simulink model "Fusion_Frame_Model_Architecture"  (R2018a)
settings: Solver=FixedStepAuto  StartTime=0.0  StopTime=SimulationTime  FixedStep=SamplingTime  RelTol=1e-3
undefined symbols (not defined in the file or in its folder): ACTIVATE_CAM, ACTIVATE_RAD, CAM1_detTimeStamp, CAM1_MeasNoise, CAM1_objClassID, CAM1_PX, CAM1_PY, CAM1_VX, CAM1_VY, CAM2_detTimeStamp, CAM2_MeasNoise, CAM2_objClassID, CAM2_PX, CAM2_PY, CAM2_VX, CAM2_VY, CAM3_detTimeStamp, CAM3_MeasNoise, CAM3_objClassID, CAM3_PX, CAM3_PY, CAM3_VX, CAM3_VY, CAM4_detTimeStamp, CAM4_MeasNoise, CAM4_objClassID, CAM4_PX, CAM4_PY, CAM4_VX, CAM4_VY, CAM5_detTimeStamp, CAM5_MeasNoise, CAM5_objClassID, CAM5_PX, CAM5_PY, CAM5_VX, CAM5_VY, CAM6_detTimeStamp, CAM6_MeasNoise, CAM6_objClassID, CAM6_PX, CAM6_PY, CAM6_VX, CAM6_VY, CAM7_detTimeStamp, CAM7_MeasNoise, CAM7_objClassID, CAM7_PX, CAM7_PY, CAM7_VX, CAM7_VY, CAM8_detTimeStamp, CAM8_MeasNoise, CAM8_objClassID, CAM8_PX, CAM8_PY, CAM8_VX, CAM8_VY, CAM_nMeas, CAM_TYPE ... (+181)
libraries: simulink_extras x4
(part 9 of 11)

== system Fusion_Frame_Model_Architecture/SENSOR_FUSION_SYSTEM/OBJECT_TRACKER_SENSOR_FUSION/RADAR_HOMOGENEOUS_FUSION/SIMPLYFIED_DBSCAN_FOR_RADAR_MEASUREMENT_GROUPING/DBSCAN_MEASUREMENT_GROUPING/COMPUTE_MEAN_IF_CLUSTER_FORMED/COMPUTE_MEAN_SUM ==
  ClusterMembers : Inport
  nPoints : Inport  Port=2
  MeasArray : Inport  Port=3
  Add1 : Sum
  Bus Selector : BusSelector  OutputSignals=MeasArray
  For Iterator : ForIterator  ResetStates=reset  IterationSource=external
  Selector : Selector  NumberOfDimensions=2  InputPortWidth=3  IndexOptions=Select all,Index vector (port)  Indices=[1 3],1  OutputSizes=1,1
  Selector1 : Selector  NumberOfDimensions=2  InputPortWidth=3  IndexOptions=Select all,Index vector (port)  Indices=[1 3],1  OutputSizes=1,1
  Unit Delay : UnitDelay  InitialCondition=single(0)  SampleTime=-1
  ClusterMeanSUM : Outport
  wires:
  nPoints/1 -> For Iterator/1
  ClusterMembers/1 -> Selector/1
  For Iterator/1 -> Selector/2
  MeasArray/1 -> Bus Selector/1
  Bus Selector/1 -> Selector1/1  "<MeasArray>"
  Selector/1 -> Selector1/2
  Selector1/1 -> Add1/2
  Unit Delay/1 -> Add1/1
  Add1/1 -> ClusterMeanSUM/1, Unit Delay/1

== system Fusion_Frame_Model_Architecture/SENSOR_FUSION_SYSTEM/OBJECT_TRACKER_SENSOR_FUSION/RADAR_HOMOGENEOUS_FUSION/SIMPLYFIED_DBSCAN_FOR_RADAR_MEASUREMENT_GROUPING/DBSCAN_MEASUREMENT_GROUPING/COMPUTE_MEAN_IF_CLUSTER_FORMED/GET_DATA ==
  CLSTR : Inport
  Bus Selector : BusSelector  OutputSignals=ClusterSizes,nClusters,ClusterMember
  Selector : Selector  NumberOfDimensions=2  InputPortWidth=3  IndexOptions=Select all,Index vector (port)  Indices=[1 3],1  OutputSizes=1,1
  nPts : Outport
  <ClusterMember> : Outport  Port=2
  wires:
  Bus Selector/1 -> Selector/1  "<ClusterSizes>"
  Selector/1 -> nPts/1
  Bus Selector/2 -> Selector/2  "<nClusters>"
  Bus Selector/3 -> <ClusterMember>/1  "<ClusterMember>"
  CLSTR/1 -> Bus Selector/1

== system Fusion_Frame_Model_Architecture/SENSOR_FUSION_SYSTEM/OBJECT_TRACKER_SENSOR_FUSION/RADAR_HOMOGENEOUS_FUSION/SIMPLYFIED_DBSCAN_FOR_RADAR_MEASUREMENT_GROUPING/DBSCAN_MEASUREMENT_GROUPING/FORM_CLUSTER/CHECK_CONDITION ==
  idx_i : Inport
  CLSTR_in : Inport  Port=2
  Bus Selector : BusSelector  OutputSignals=isMeasVisitedFlag
  Logical Operator1 : Logic  Operator=NOT  AllPortsSameDT=off  OutDataTypeStr=boolean
  Selector1 : Selector  NumberOfDimensions=2  InputPortWidth=3  IndexOptions=Select all,Index vector (port)  Indices=1,1  OutputSizes=1,1
  Unit Delay : UnitDelay  InitialCondition=CLSTR_SNSR_DELAY_INIT  SampleTime=-1
  isNotVisited : Outport
  CLSTR_out : Outport  Port=2
  wires:
  Logical Operator1/1 -> isNotVisited/1
  Selector1/1 -> Logical Operator1/1
  idx_i/1 -> Selector1/2
  CLSTR_in/1 -> Unit Delay/1
  Bus Selector/1 -> Selector1/1  "<isMeasVisitedFlag>"
  Unit Delay/1 -> CLSTR_out/1, Bus Selector/1

== system Fusion_Frame_Model_Architecture/SENSOR_FUSION_SYSTEM/OBJECT_TRACKER_SENSOR_FUSION/RADAR_HOMOGENEOUS_FUSION/SIMPLYFIED_DBSCAN_FOR_RADAR_MEASUREMENT_GROUPING/DBSCAN_MEASUREMENT_GROUPING/FORM_CLUSTER/DBSCAN ==
  CLSTR_DATA : Inport
  measArray : Inport  Port=2
  idx_i : Inport  Port=3
  Action Port : ActionPort  ActionType=then
  DBSCAN_PROPAGATE_AND_EXPAND_CLUSTER : Subsystem
  INITIALIZE_CLUSTER : Subsystem
  Subsystem : Subsystem
  nPtsEps : Outport
  CLSTR_DATA_UPD : Outport  Port=2
  wires:
  idx_i/1 -> INITIALIZE_CLUSTER/3(idx_i)
  INITIALIZE_CLUSTER/2(CLUSTER_DATA) -> DBSCAN_PROPAGATE_AND_EXPAND_CLUSTER/3(CLSTR_DATA)
  INITIALIZE_CLUSTER/1(nRadMeas) -> DBSCAN_PROPAGATE_AND_EXPAND_CLUSTER/1(nMeas)
  CLSTR_DATA/1 -> INITIALIZE_CLUSTER/1(CLUSTERING_DATA)
  [meas] -> DBSCAN_PROPAGATE_AND_EXPAND_CLUSTER/2(measArray)
  measArray/1 -> INITIALIZE_CLUSTER/2(RAD_MEAS_CTS), [meas]
  DBSCAN_PROPAGATE_AND_EXPAND_CLUSTER/1(CLSTR_DATA_UPD) -> CLSTR_DATA_UPD/1, Subsystem/1(CLSTR_DATA)
  Subsystem/1(ClstrSize) -> nPtsEps/1

== system Fusion_Frame_Model_Architecture/SENSOR_FUSION_SYSTEM/OBJECT_TRACKER_SENSOR_FUSION/RADAR_HOMOGENEOUS_FUSION/SIMPLYFIED_DBSCAN_FOR_RADAR_MEASUREMENT_GROUPING/DBSCAN_MEASUREMENT_GROUPING/FORM_CLUSTER/MERGE_SIGNALS ==
  CLSTR_NO_UPD : Inport
  nPtsEpsNoUpd : Inport  Port=2
  nPtsUpd : Inport  Port=3
  CLSTR_UPD : Inport  Port=4
  Merge : Merge
  Merge1 : Merge
  nPtsEps : Outport
  CLSTR_DATA : Outport  Port=2
  wires:
  CLSTR_NO_UPD/1 -> Merge1/1
  Merge1/1 -> CLSTR_DATA/1
  nPtsEpsNoUpd/1 -> Merge/1
  Merge/1 -> nPtsEps/1
  nPtsUpd/1 -> Merge/2
  CLSTR_UPD/1 -> Merge1/2

== system Fusion_Frame_Model_Architecture/SENSOR_FUSION_SYSTEM/OBJECT_TRACKER_SENSOR_FUSION/RADAR_HOMOGENEOUS_FUSION/SIMPLYFIED_DBSCAN_FOR_RADAR_MEASUREMENT_GROUPING/DBSCAN_MEASUREMENT_GROUPING/FORM_CLUSTER/NO_CLUSTER_FORMED ==
  CLSTR_DATA : Inport
  Action Port : ActionPort  ActionType=else
  Constant : Constant  Value=uint16(0)
  CLSTR_DATA_NO_UPD : Outport
  nPtsEpsNoUpd : Outport  Port=2
  wires:
  CLSTR_DATA/1 -> CLSTR_DATA_NO_UPD/1
  Constant/1 -> nPtsEpsNoUpd/1

== system Fusion_Frame_Model_Architecture/SENSOR_FUSION_SYSTEM/OBJECT_TRACKER_SENSOR_FUSION/RADAR_HOMOGENEOUS_FUSION/SIMPLYFIED_DBSCAN_FOR_RADAR_MEASUREMENT_GROUPING/DBSCAN_MEASUREMENT_GROUPING/MERGE_SIGNALS/GET_DATA_FROM_BUS ==
  CLSTR_DATA : Inport
  Bus Selector : BusSelector  OutputSignals=ClusterCenter,ClusterCovariance,nClusters
  <ClusterCenter> : Outport
  <ClusterCovariance> : Outport  Port=2
  <nClusters> : Outport  Port=3
  wires:
  Bus Selector/3 -> <nClusters>/1  "<nClusters>"
  Bus Selector/1 -> <ClusterCenter>/1  "<ClusterCenter>"
  CLSTR_DATA/1 -> Bus Selector/1
  Bus Selector/2 -> <ClusterCovariance>/1  "<ClusterCovariance>"

== system Fusion_Frame_Model_Architecture/SENSOR_FUSION_SYSTEM/OBJECT_TRACKER_SENSOR_FUSION/RADAR_HOMOGENEOUS_FUSION/SIMPLYFIED_DBSCAN_FOR_RADAR_MEASUREMENT_GROUPING/DBSCAN_MEASUREMENT_GROUPING/MERGE_SIGNALS/SET_DATA_TO_BUS ==
  CLSTR_DATA : Inport
  Mean_ARRAY : Inport  Port=2
  Cov_ARRAY : Inport  Port=3
  Bus Creator : BusCreator  Inputs=7  OutDataTypeStr=Bus: CLUSTER_DATA_STRUCT_SNSR  NonVirtualBus=on
      settings: InheritFromInputs=off
  Bus Selector1 : BusSelector  OutputSignals=ClusterCenter,ClusterCovariance,ClusterSizes,ClusterToMeasAssignment,isMeasVisitedFlag,nClusters,ClusterMember
  Constant1 : Constant  Value=ClusterMemArray_SNSR
  Reshape1 : Reshape  OutputDimensionality=Row vector (2-D)
  Terminator1 : Terminator
  Terminator2 : Terminator
  Terminator3 : Terminator
  "CLSTR_DATA_UPD " : Outport
  wires:
  Constant1/1 -> Reshape1/1  "ClusterMember"
  Bus Selector1/5 -> Bus Creator/5  "<isMeasVisitedFlag>"
  Cov_ARRAY/1 -> Bus Creator/2  "ClusterCovariance"
  Mean_ARRAY/1 -> Bus Creator/1  "ClusterCenter"
  Bus Selector1/1 -> Terminator2/1  "<ClusterCenter>"
  Bus Selector1/7 -> Terminator1/1  "<ClusterMember>"
  Bus Selector1/2 -> Terminator3/1  "<ClusterCovariance>"
  Bus Selector1/3 -> Bus Creator/3  "<ClusterSizes>"
  Reshape1/1 -> Bus Creator/7  "ClusterMember"
  Bus Selector1/4 -> Bus Creator/4  "<ClusterToMeasAssignment>"
  Bus Selector1/6 -> Bus Creator/6  "<nClusters>"
  Bus Creator/1 -> "CLSTR_DATA_UPD "/1
  CLSTR_DATA/1 -> Bus Selector1/1

== system Fusion_Frame_Model_Architecture/SENSOR_FUSION_SYSTEM/OBJECT_TRACKER_SENSOR_FUSION/RADAR_HOMOGENEOUS_FUSION/SIMPLYFIED_DBSCAN_FOR_RADAR_MEASUREMENT_GROUPING/DBSCAN_MEASUREMENT_GROUPING/MERGE_SIGNALS/UPDATE_CLUSTER_DATA ==
  Center_ARRAY : Inport
  Cov_ARRAY : Inport  Port=2
  ID : Inport  Port=3
  mean1 : Inport  Port=4
  mean2 : Inport  Port=5
  Cov1 : Inport  Port=6
  Cov2 : Inport  Port=7
  FLAG : Inport  Port=8
  Assignment : Assignment  NumberOfDimensions=2  DiagnosticForDimensions=Warning  IndexOptions=Assign all,Index vector (port)  Indices=1,1  OutputSizes=1,1
  Assignment1 : Assignment  NumberOfDimensions=3  DiagnosticForDimensions=Warning  IndexOptions=Assign all,Assign all,Index vector (port)  Indices=1,1,1  OutputSizes=1,1,1
  Merge : Merge
  Merge2 : Merge
  Selector : Selector  NumberOfDimensions=2  InputPortWidth=3  IndexOptions=Select all,Index vector (port)  Indices=[1 3],1  OutputSizes=1,1
  Selector1 : Selector  NumberOfDimensions=3  InputPortWidth=3  IndexOptions=Select all,Select all,Index vector (port)  Indices=[1 3],1,1  OutputSizes=1,1,1
  Switch : Switch  Criteria=u2 ~= 0
  Switch1 : Switch  Criteria=u2 ~= 0
  CenterUpd : Outport
  CovUpd : Outport  Port=2
  wires:
  Selector/1 -> Switch/3
  Merge2/1 -> Switch1/1
  Cov_ARRAY/1 -> Assignment1/1, Selector1/1
  mean1/1 -> Merge/1
  Selector1/1 -> Switch1/3
  Merge/1 -> Switch/1
  Switch1/1 -> Assignment1/2
  Switch/1 -> Assignment/2
  Cov2/1 -> Merge2/2
  Assignment1/1 -> CovUpd/1
  Assignment/1 -> CenterUpd/1
  Cov1/1 -> Merge2/1
  mean2/1 -> Merge/2
  FLAG/1 -> [FLAG]
  [FLAG] -> Switch/2
  [FLAG] -> Switch1/2
  [ID] -> Assignment/3, Selector/2
  ID/1 -> [ID], Assignment1/3, Selector1/2
  Center_ARRAY/1 -> Selector/1, Assignment/1

== system Fusion_Frame_Model_Architecture/SENSOR_FUSION_SYSTEM/OBJECT_TRACKER_SENSOR_FUSION/SENSOR_LAYOUT_AND_CHRACTERIZATION/PRE_COMPUTE_SENSOR_FOV_GRID/COMPUTE_CAMERA_SNSR_GRID/ComputeCoverageANDConfidence/Compute_Cell_X_and_Y_index ==
  CellIndex : Inport
  GridID_vec : Inport  Port=2
  GridParam : Inport  Port=3
  SensorExtrinsicParam : Inport  Port=4
  SensorIntrinsicParam : Inport  Port=5
  Compute_Cell_X_Y_Center_Coordinate : Subsystem
  Compute_FOV_Overlap_with_Cell_and_Region_Confidence : Subsystem
  GET_DATA : Subsystem
  Transform_Cell_Coordinate_Vehicle_Frame_To_Sensor_Frame : Subsystem
  RegionConfidence : Outport
  FOVOverlap : Outport  Port=2
  wires:
  GridID_vec/1 -> GET_DATA/1(GridID_vector)
  CellIndex/1 -> GET_DATA/2(index)
  GridParam/1 -> GET_DATA/3(GridParam)
  GET_DATA/1(CellID) -> Compute_Cell_X_Y_Center_Coordinate/1(Cell_id)
  GET_DATA/2(<xRes>) -> Compute_Cell_X_Y_Center_Coordinate/2(xRes)
  GET_DATA/3(<xRear>) -> Compute_Cell_X_Y_Center_Coordinate/3(xRear)
  GET_DATA/4(<nGridCellsLat>) -> Compute_Cell_X_Y_Center_Coordinate/4(Cy)
  GET_DATA/5(<yRes>) -> Compute_Cell_X_Y_Center_Coordinate/5(yRes)
  GET_DATA/6(<yLeft>) -> Compute_Cell_X_Y_Center_Coordinate/6(yLeft)
  SensorExtrinsicParam/1 -> Transform_Cell_Coordinate_Vehicle_Frame_To_Sensor_Frame/3(SensorExtrinsic)
  Compute_Cell_X_Y_Center_Coordinate/1(CellCenterCoordX) -> Transform_Cell_Coordinate_Vehicle_Frame_To_Sensor_Frame/1(Cell_xCoord)
  Compute_Cell_X_Y_Center_Coordinate/2(CellCenterCoordY) -> Transform_Cell_Coordinate_Vehicle_Frame_To_Sensor_Frame/2(Cell_y_Coord)
  Transform_Cell_Coordinate_Vehicle_Frame_To_Sensor_Frame/1(Cell_xSnsrCoord) -> Compute_FOV_Overlap_with_Cell_and_Region_Confidence/1(Cell_xSnsrCoord)
  Transform_Cell_Coordinate_Vehicle_Frame_To_Sensor_Frame/2(Cell_ySnsrCoord) -> Compute_FOV_Overlap_with_Cell_and_Region_Confidence/2(Cell_ySnsrCoord)
  SensorIntrinsicParam/1 -> Compute_FOV_Overlap_with_Cell_and_Region_Confidence/3(SnsrIntrinsic)
  Compute_FOV_Overlap_with_Cell_and_Region_Confidence/1(RegionConfidence) -> RegionConfidence/1
  Compute_FOV_Overlap_with_Cell_and_Region_Confidence/2(FOVOverlap) -> FOVOverlap/1

== system Fusion_Frame_Model_Architecture/SENSOR_FUSION_SYSTEM/OBJECT_TRACKER_SENSOR_FUSION/SENSOR_LAYOUT_AND_CHRACTERIZATION/PRE_COMPUTE_SENSOR_FOV_GRID/COMPUTE_CAMERA_SNSR_GRID/ComputeCoverageANDConfidence/SET_DATA ==
  GridIndex : Inport
  RegionConfiArray : Inport  Port=2
  FOVOverlapArray : Inport  Port=3
  SnsrIndex : Inport  Port=4
  confi : Inport  Port=5
  overlap : Inport  Port=6
  Assignment : Assignment  NumberOfDimensions=2  DiagnosticForDimensions=Warning  IndexOptions=Index vector (port),Index vector (port)  Indices=1,1  OutputSizes=1,1
  Assignment1 : Assignment  NumberOfDimensions=2  DiagnosticForDimensions=Warning  IndexOptions=Index vector (port),Index vector (port)  Indices=1,1  OutputSizes=1,1
  RegionConfidence : Outport
  FOVOverlap : Outport  Port=2
  wires:
  SnsrIndex/1 -> Assignment1/3, Assignment/3
  RegionConfiArray/1 -> Assignment/1
  Assignment/1 -> RegionConfidence/1
  GridIndex/1 -> Assignment/4, Assignment1/4
  Assignment1/1 -> FOVOverlap/1
  overlap/1 -> Assignment1/2
  FOVOverlapArray/1 -> Assignment1/1
  confi/1 -> Assignment/2

== system Fusion_Frame_Model_Architecture/SENSOR_FUSION_SYSTEM/OBJECT_TRACKER_SENSOR_FUSION/SENSOR_LAYOUT_AND_CHRACTERIZATION/PRE_COMPUTE_SENSOR_FOV_GRID/COMPUTE_RADAR_SNSR_GRID/ComputeCoverageANDConfidence/Compute_Cell_X_and_Y_index ==
  CellIndex : Inport
  GridID_vec : Inport  Port=2
  GridParam : Inport  Port=3
  SensorExtrinsicParam : Inport  Port=4
  SensorIntrinsicParam : Inport  Port=5
  Compute_Cell_X_Y_Center_Coordinate : Subsystem
  Compute_FOV_Overlap_with_Cell_and_Region_Confidence : Subsystem
  GET_DATA : Subsystem
  Transform_Cell_Coordinate_Vehicle_Frame_To_Sensor_Frame : Subsystem
  RegionConfidence : Outport
  FOVOverlap : Outport  Port=2
  wires:
  GridID_vec/1 -> GET_DATA/1(GridID_vector)
  CellIndex/1 -> GET_DATA/2(index)
  GridParam/1 -> GET_DATA/3(GridParam)
  GET_DATA/1(CellID) -> Compute_Cell_X_Y_Center_Coordinate/1(Cell_id)
  GET_DATA/2(<xRes>) -> Compute_Cell_X_Y_Center_Coordinate/2(xRes)
  GET_DATA/3(<xRear>) -> Compute_Cell_X_Y_Center_Coordinate/3(xRear)
  GET_DATA/4(<nGridCellsLat>) -> Compute_Cell_X_Y_Center_Coordinate/4(Cy)
  GET_DATA/5(<yRes>) -> Compute_Cell_X_Y_Center_Coordinate/5(yRes)
  GET_DATA/6(<yLeft>) -> Compute_Cell_X_Y_Center_Coordinate/6(yLeft)
  SensorExtrinsicParam/1 -> Transform_Cell_Coordinate_Vehicle_Frame_To_Sensor_Frame/3(SensorExtrinsic)
  Compute_Cell_X_Y_Center_Coordinate/1(CellCenterCoordX) -> Transform_Cell_Coordinate_Vehicle_Frame_To_Sensor_Frame/1(Cell_xCoord)
  Compute_Cell_X_Y_Center_Coordinate/2(CellCenterCoordY) -> Transform_Cell_Coordinate_Vehicle_Frame_To_Sensor_Frame/2(Cell_y_Coord)
  Transform_Cell_Coordinate_Vehicle_Frame_To_Sensor_Frame/1(Cell_xSnsrCoord) -> Compute_FOV_Overlap_with_Cell_and_Region_Confidence/1(Cell_xSnsrCoord)
  Transform_Cell_Coordinate_Vehicle_Frame_To_Sensor_Frame/2(Cell_ySnsrCoord) -> Compute_FOV_Overlap_with_Cell_and_Region_Confidence/2(Cell_ySnsrCoord)
  SensorIntrinsicParam/1 -> Compute_FOV_Overlap_with_Cell_and_Region_Confidence/3(SnsrIntrinsic)
  Compute_FOV_Overlap_with_Cell_and_Region_Confidence/1(RegionConfidence) -> RegionConfidence/1
  Compute_FOV_Overlap_with_Cell_and_Region_Confidence/2(FOVOverlap) -> FOVOverlap/1

== system Fusion_Frame_Model_Architecture/SENSOR_FUSION_SYSTEM/OBJECT_TRACKER_SENSOR_FUSION/SENSOR_LAYOUT_AND_CHRACTERIZATION/PRE_COMPUTE_SENSOR_FOV_GRID/COMPUTE_RADAR_SNSR_GRID/ComputeCoverageANDConfidence/SET_DATA ==
  GridIndex : Inport
  RegionConfiArray : Inport  Port=2
  FOVOverlapArray : Inport  Port=3
  SnsrIndex : Inport  Port=4
  confi : Inport  Port=5
  overlap : Inport  Port=6
  Assignment : Assignment  NumberOfDimensions=2  DiagnosticForDimensions=Warning  IndexOptions=Index vector (port),Index vector (port)  Indices=1,1  OutputSizes=1,1
  Assignment1 : Assignment  NumberOfDimensions=2  DiagnosticForDimensions=Warning  IndexOptions=Index vector (port),Index vector (port)  Indices=1,1  OutputSizes=1,1
  RegionConfidence : Outport
  FOVOverlap : Outport  Port=2
  wires:
  SnsrIndex/1 -> Assignment1/3, Assignment/3
  RegionConfiArray/1 -> Assignment/1
  Assignment/1 -> RegionConfidence/1
  GridIndex/1 -> Assignment/4, Assignment1/4
  Assignment1/1 -> FOVOverlap/1
  overlap/1 -> Assignment1/2
  FOVOverlapArray/1 -> Assignment1/1
  confi/1 -> Assignment/2

== system Fusion_Frame_Model_Architecture/SENSOR_FUSION_SYSTEM/OBJECT_TRACKER_SENSOR_FUSION/SENSOR_LAYOUT_AND_CHRACTERIZATION/PRE_COMPUTE_SENSOR_FOV_GRID/CREATE_GRID/For Iterator Subsystem/Compute_Grid_Cell_Cartesian_Coordinate ==
  note: Get_Grid_Limits_Data
  note: Compute_Grid_Cell_x_Coordinate
  note: Compute_Grid_Cell_y_Coordinate
  GridParam : Inport
  x_Index : Inport  Port=2
  y_Index : Inport  Port=3
  Add : Sum
  Add1 : Sum
  Bus Selector : BusSelector  OutputSignals=xRes,xRear
  Bus Selector1 : BusSelector  OutputSignals=yRes,yLeft
  Bus Selector2 : BusSelector  OutputSignals=xGridParameters,yGridParameters
  Constant : Constant  Value=single(1)
  Multiply : Product
  Multiply1 : Product
  Subtract : Sum  Inputs=+-
  Subtract1 : Sum  Inputs=-+
  x_Coordinate : Outport
  y_Coordinate : Outport  Port=2
  wires:
  [xRes] -> Multiply/2
  Add/1 -> x_Coordinate/1
  Subtract/1 -> Multiply/1
  Constant/1 -> Subtract/2, Subtract1/1
  [xRear] -> Add/2
  Multiply/1 -> Add/1
  [yRes] -> Multiply1/2
  y_Index/1 -> Subtract1/2
  Add1/1 -> y_Coordinate/1
  Multiply1/1 -> Add1/1
  Subtract1/1 -> Multiply1/1
  [yLeft] -> Add1/2
  Bus Selector/1 -> [xRes]  "<xRes>"
  Bus Selector1/1 -> [yRes]  "<yRes>"
  Bus Selector1/2 -> [yLeft]  "<yLeft>"
  Bus Selector/2 -> [xRear]  "<xRear>"
  x_Index/1 -> Subtract/1
  Bus Selector2/1 -> Bus Selector/1  "<xGridParameters>"
  GridParam/1 -> Bus Selector2/1
  Bus Selector2/2 -> Bus Selector1/1  "<yGridParameters>"

== system Fusion_Frame_Model_Architecture/SENSOR_FUSION_SYSTEM/OBJECT_TRACKER_SENSOR_FUSION/SENSOR_LAYOUT_AND_CHRACTERIZATION/PRE_COMPUTE_SENSOR_FOV_GRID/CREATE_GRID/For Iterator Subsystem/Compute_Grid_Cell_Discreete_Index ==
  note: Get_Data
  note: 2D_Cell_Index_To_1D_Cell_Index
  note: Compute_Grid_X_Index
  note: Compute_x_index
  note: Compute_x_index_Lower_Limit
  note: Translate_x_index_to_make_it_positive
  note: Compute_Grid_Y_Index
  note: Compute_y_index
  note: Translate_y_index_to_make_it_positive
  note: Compute_y_index_Lower_Limit
  GridParam : Inport
  x_coord : Inport  Port=2
  y_coord : Inport  Port=3
  Add : Sum
  Bus Selector : BusSelector  OutputSignals=xRes,xRear
  Bus Selector1 : BusSelector  OutputSignals=nGridCellsLat,yRes,yLeft
  Bus Selector2 : BusSelector  OutputSignals=xGridParameters,yGridParameters
  Divide : Product  Inputs=*/
  Divide1 : Product  Inputs=*/
  Divide2 : Product  Inputs=/*
  Divide3 : Product  Inputs=/*
  Floor{,1..3} (4 alike) : Rounding
  Minus : Sum  Inputs=+-
  Minus1 : Sum  Inputs=+-
  Multiply : Product
  CellID_x : Outport
  CellID_y : Outport  Port=2
  CellID : Outport  Port=3
  wires:
  Minus/1 -> Multiply/1, CellID_x/1
  Floor/1 -> Minus/1
  Floor2/1 -> Minus/2
  Divide/1 -> Floor/1
  Divide2/1 -> Floor2/1
  x_coord/1 -> Divide/1
  [xRes] -> Divide2/1, Divide/2
  [xRear] -> Divide2/2
  y_coord/1 -> Divide1/1
  [yRes] -> Divide3/1, Divide1/2
  [yLeft] -> Divide3/2
  Floor3/1 -> Minus1/2
  Divide3/1 -> Floor3/1
  Divide1/1 -> Floor1/1
  Floor1/1 -> Minus1/1
  Minus1/1 -> Add/2, CellID_y/1
  [Cy] -> Multiply/2
  Multiply/1 -> Add/1
  Add/1 -> CellID/1
  Bus Selector/2 -> [xRear]  "<xRear>"
  Bus Selector2/1 -> Bus Selector/1  "<xGridParameters>"
  GridParam/1 -> Bus Selector2/1
  Bus Selector2/2 -> Bus Selector1/1  "<yGridParameters>"
  Bus Selector/1 -> [xRes]  "<xRes>"
  Bus Selector1/3 -> [yLeft]  "<yLeft>"
  Bus Selector1/2 -> [yRes]  "<yRes>"
  Bus Selector1/1 -> [Cy]  "<nGridCellsLat>"

== system Fusion_Frame_Model_Architecture/SENSOR_FUSION_SYSTEM/OBJECT_TRACKER_SENSOR_FUSION/SENSOR_LAYOUT_AND_CHRACTERIZATION/PRE_COMPUTE_SENSOR_FOV_GRID/CREATE_GRID/For Iterator Subsystem/SET_DATA ==
  CellIDArray : Inport
  CellID : Inport  Port=2
  Assignment : Assignment  NumberOfDimensions=2  DiagnosticForDimensions=Warning  IndexOptions=Assign all,Index vector (port)  Indices=1,1  OutputSizes=1,1
  Constant2 : Constant  Value=int32(1)
  Data Type Conversion1 : DataTypeConversion  OutDataTypeStr=int32
  Data Type Conversion3 : DataTypeConversion  OutDataTypeStr=int32
  Reshape : Reshape  OutputDimensionality=Row vector (2-D)
  Subtract : Sum
  CellIDArrayUpd : Outport
  wires:
  CellIDArray/1 -> Reshape/1
  Assignment/1 -> CellIDArrayUpd/1
  Constant2/1 -> Subtract/2
  CellID/1 -> Data Type Conversion1/1, Assignment/2
  Data Type Conversion3/1 -> Assignment/3
  Data Type Conversion1/1 -> Subtract/1
  Subtract/1 -> Data Type Conversion3/1
  Reshape/1 -> Assignment/1

== system Fusion_Frame_Model_Architecture/SENSOR_FUSION_SYSTEM/OBJECT_TRACKER_SENSOR_FUSION/SENSOR_LAYOUT_AND_CHRACTERIZATION/SET_SENSOR_CALLIBRATION_PARAMETER/SET_CAMERA_SENSOR_PARAM/SET_CAMERA_EXTRINSIC_PARAM/SET_CAMERA_EXTRINSIC_PARAM ==
  SensorParam : Inport
  SensorID : Inport  Port=2
  Assignment : Assignment  DiagnosticForDimensions=Warning  IndexOptions=Index vector (port)  Indices=1  OutputSizes=1
  Bus Creator : BusCreator  Inputs=12  OutDataTypeStr=Bus: CameraExtrinsicParam  NonVirtualBus=on
  Bus Selector : BusSelector  OutputSignals=CameraID,CameraType,isActive,RotMat2D,TranslationVec,MountX,MountY,MountZ,MountYaw,MountPitch,MountRoll,nMeas
  Constant : Constant  Value=ACTIVATE_CAM
  Constant1 : Constant  Value=CAM_X_INSTALL
  Constant2 : Constant  Value=CAM_Y_INSTALL
  Constant3 : Constant  Value=CAM_YAW_INSTALL
  Constant4 : Constant  Value=CAM_nMeas
  Constant9 : Constant  Value=CAM_TYPE
  CreateRotationMatTranslationVector : Subsystem
  Data Type Conversion : DataTypeConversion  OutDataTypeStr=uint8
  Selector{,1..5,8} (7 alike) : Selector  InputPortWidth=nCameras  IndexOptions=Index vector (port)  Indices=[1 3]  OutputSizes=1
  Terminator{,1..8} (9 alike) : Terminator
  Out1 : Outport
  wires:
  Assignment/1 -> Out1/1
  Constant/1 -> Selector1/1
  SensorParam/1 -> [Param], Selector/1
  Constant2/1 -> Selector3/1
  [SensorID] -> Selector5/2, Selector4/2, Selector3/2, Selector2/2, Selector1/2, Selector8/2, Data Type Conversion/1
  Constant3/1 -> Selector4/1
  Constant1/1 -> Selector2/1
  Selector/1 -> Bus Selector/1
  Bus Creator/1 -> Assignment/2
  Bus Selector/1 -> Terminator/1  "<CameraID>"
  SensorID/1 -> [SensorID], Selector/2
  [Param] -> Assignment/1
  [SensorID] -> Assignment/3
  Selector2/1 -> [MountX], Bus Creator/6  "MountX"
  Selector3/1 -> [MountY], Bus Creator/7  "MountY"
  [MountX] -> CreateRotationMatTranslationVector/2(xMount)
  [MountY] -> CreateRotationMatTranslationVector/3(yMount)
  Selector4/1 -> [MountYaw], Bus Creator/9  "MountYaw"
  [MountYaw] -> CreateRotationMatTranslationVector/1(yawInstall)
  CreateRotationMatTranslationVector/1(RotMatrx) -> [RotMat]
  CreateRotationMatTranslationVector/2(TranslationVector) -> [TransVec]
  Data Type Conversion/1 -> Bus Creator/1  "CameraID"
  Selector8/1 -> Bus Creator/2  "CameraType"
  Constant9/1 -> Selector8/1
  Selector1/1 -> Bus Creator/3  "isActive"
  [RotMat] -> Bus Creator/4  "RotMat2D"
  [TransVec] -> Bus Creator/5  "TranslationVec"
  Bus Selector/2 -> Terminator1/1  "<CameraType>"
  Bus Selector/3 -> Terminator2/1  "<isActive>"
  Bus Selector/4 -> Terminator3/1  "<RotMat2D>"
  Bus Selector/8 -> Bus Creator/8  "<MountZ>"
  Bus Selector/5 -> Terminator4/1  "<TranslationVec>"
  Bus Selector/7 -> Terminator6/1  "<MountY>"
  Bus Selector/6 -> Terminator5/1  "<MountX>"
  Bus Selector/9 -> Terminator8/1  "<MountYaw>"
  Bus Selector/11 -> Bus Creator/11  "<MountRoll>"
  Bus Selector/10 -> Bus Creator/10  "<MountPitch>"
  Selector5/1 -> Bus Creator/12  "nMeas"
  Constant4/1 -> Selector5/1
  Bus Selector/12 -> Terminator7/1  "<nMeas>"

== system Fusion_Frame_Model_Architecture/SENSOR_FUSION_SYSTEM/OBJECT_TRACKER_SENSOR_FUSION/SENSOR_LAYOUT_AND_CHRACTERIZATION/SET_SENSOR_CALLIBRATION_PARAMETER/SET_CAMERA_SENSOR_PARAM/SET_CAMERA_INTRINSIC_PARAM/SET_CAMERA_INTRINSIC_PARAM ==
  SensorParam : Inport
  SensorID : Inport  Port=2
  Assignment : Assignment  DiagnosticForDimensions=Warning  IndexOptions=Index vector (port)  Indices=1  OutputSizes=1
  Bus Creator : BusCreator  Inputs=12  OutDataTypeStr=Bus: CameraIntrinsicParam  NonVirtualBus=on
  Bus Selector : BusSelector  OutputSignals=CameraType,RectificationMatrix,ProjectionMatrix,MaxRange,MaxAzimuth,MaxElevation,LongitudinalErrVariance,LateralErrVariance,ProbOfDetection,FalseAlarmRate,FOVRangePoints,FOVAzimuthPts
  Constant1 : Constant  Value=CAMERA_LONG_ERR_VAR
  Constant15 : Constant  Value=RADAR_PD
  Constant16 : Constant  Value=RADAR_FA
  Constant2 : Constant  Value=CAMERA_MAX_ELEVATION
  Constant3 : Constant  Value=CAMERA_LAT_ERR_VAR
  Constant4 : Constant  Value=CAMERA_MAX_RANGE
  Constant5 : Constant  Value=CAMERA_MAX_AZIMUTH
  Data Type Conversion : DataTypeConversion  OutDataTypeStr=uint8
  Selector{,1..3,5..6} (6 alike) : Selector  InputPortWidth=nCameraTypes  IndexOptions=Index vector (port)  Indices=[1 3]  OutputSizes=1
  Selector14 : Selector  InputPortWidth=nRadarTypes  IndexOptions=Index vector (port)  Indices=[1 3]  OutputSizes=1
  Selector15 : Selector  InputPortWidth=nRadarTypes  IndexOptions=Index vector (port)  Indices=[1 3]  OutputSizes=1
  Terminator{,1..7} (8 alike) : Terminator
  Out1 : Outport
  wires:
  Assignment/1 -> Out1/1
  SensorParam/1 -> [Param], Selector/1
  Selector/1 -> Bus Selector/1
  Bus Creator/1 -> Assignment/2
  SensorID/1 -> Selector/2, [SnsrTypeID]
  [Param] -> Assignment/1
  [SnsrTypeID] -> Assignment/3
  Constant5/1 -> Selector6/1
  Constant4/1 -> Selector5/1
  [SnsrTypeID] -> Selector15/2, Selector14/2, Selector3/2, Selector2/2, Selector1/2, Selector6/2, Selector5/2, Data Type Conversion/1
  Constant2/1 -> Selector1/1
  Constant15/1 -> Selector14/1
  Constant16/1 -> Selector15/1
  Bus Selector/1 -> Terminator/1  "<CameraType>"
  Bus Selector/2 -> Bus Creator/2  "<RectificationMatrix>"
  Bus Selector/4 -> Terminator3/1  "<MaxRange>"
  Bus Selector/3 -> Bus Creator/3  "<ProjectionMatrix>"
  Bus Selector/6 -> Terminator5/1  "<MaxElevation>"
  Bus Selector/7 -> Terminator6/1  "<LongitudinalErrVariance>"
  Bus Selector/8 -> Terminator7/1  "<LateralErrVariance>"
  Bus Selector/5 -> Terminator4/1  "<MaxAzimuth>"
  Selector5/1 -> Bus Creator/4  "MaxRange"
  Selector6/1 -> Bus Creator/5  "MaxAzimuth"
  Selector1/1 -> Bus Creator/6  "MaxElevation"
  Selector2/1 -> Bus Creator/7  "LongitudinalErrVariance"
  Selector3/1 -> Bus Creator/8  "LateralErrVariance"
  Constant1/1 -> Selector2/1
  Constant3/1 -> Selector3/1
  Selector14/1 -> Bus Creator/9  "ProbOfDetection"
  Selector15/1 -> Bus Creator/10  "FalseAlarmRate"
  Bus Selector/11 -> Bus Creator/11  "<FOVRangePoints>"
  Bus Selector/12 -> Bus Creator/12  "<FOVAzimuthPts>"
  Bus Selector/9 -> Terminator1/1  "<ProbOfDetection>"
  Bus Selector/10 -> Terminator2/1  "<FalseAlarmRate>"
  Data Type Conversion/1 -> Bus Creator/1  "CameraType"

== system Fusion_Frame_Model_Architecture/SENSOR_FUSION_SYSTEM/OBJECT_TRACKER_SENSOR_FUSION/SENSOR_LAYOUT_AND_CHRACTERIZATION/SET_SENSOR_CALLIBRATION_PARAMETER/SET_RADAR_SENSOR_PARAM/SET_RADAR_EXTRINSIC_PARAM/SET_RADAR_EXTRINSIC_PARAM ==
  SensorParam : Inport
  SensorID : Inport  Port=2
  Assignment : Assignment  DiagnosticForDimensions=Warning  IndexOptions=Index vector (port)  Indices=1  OutputSizes=1
  Bus Creator : BusCreator  Inputs=12  OutDataTypeStr=Bus: RadarExtrinsicParam  NonVirtualBus=on
  Bus Selector : BusSelector  OutputSignals=RadarID,RadarType,isActive,RotMat2D,TranslationVec,MountX,MountY,MountZ,MountYaw,MountPitch,MountRoll,nMeas
  CREATE_ROTATION_MATRIX_TRANSLATION_VECTOR : Subsystem
  Constant : Constant  Value=ACTIVATE_RAD
  Constant1 : Constant  Value=RAD_X_INSTALL
  Constant2 : Constant  Value=RAD_Y_INSTALL
  Constant3 : Constant  Value=RAD_YAW_INSTALL
  Constant4 : Constant  Value=RAD_nMeas
  Constant9 : Constant  Value=RAD_TYPE
  Data Type Conversion : DataTypeConversion  OutDataTypeStr=uint8
  Selector{,1..5,8} (7 alike) : Selector  InputPortWidth=nRadars  IndexOptions=Index vector (port)  Indices=[1 3]  OutputSizes=1
  Terminator{,1..8} (9 alike) : Terminator
  RadarSensorParam : Outport
  wires:
  Assignment/1 -> RadarSensorParam/1
  Constant/1 -> Selector1/1
  SensorParam/1 -> [Param], Selector/1
  Constant2/1 -> Selector3/1
  [SensorID] -> Selector5/2, Selector4/2, Selector3/2, Selector2/2, Selector1/2, Selector8/2, Data Type Conversion/1
  Constant3/1 -> Selector4/1
  Constant1/1 -> Selector2/1
  Selector/1 -> Bus Selector/1
  Bus Creator/1 -> Assignment/2
  Bus Selector/1 -> Terminator/1  "<RadarID>"
  SensorID/1 -> [SensorID], Selector/2
  [Param] -> Assignment/1
  [SensorID] -> Assignment/3
  Selector2/1 -> [MountX], Bus Creator/6  "MountX"
  Selector3/1 -> [MountY], Bus Creator/7  "MountY"
  [MountX] -> CREATE_ROTATION_MATRIX_TRANSLATION_VECTOR/2(xMount)
  [MountY] -> CREATE_ROTATION_MATRIX_TRANSLATION_VECTOR/3(yMount)
  Selector4/1 -> [MountYaw], Bus Creator/9  "MountYaw"
  [MountYaw] -> CREATE_ROTATION_MATRIX_TRANSLATION_VECTOR/1(yawInstall)
  CREATE_ROTATION_MATRIX_TRANSLATION_VECTOR/1(RotMatrx) -> [RotMat]
  CREATE_ROTATION_MATRIX_TRANSLATION_VECTOR/2(TranslationVector) -> [TransVec]
  Data Type Conversion/1 -> Bus Creator/1  "RadarID"
  Selector8/1 -> Bus Creator/2  "RadarType"
  Constant9/1 -> Selector8/1
  Selector1/1 -> Bus Creator/3  "isActive"
  [RotMat] -> Bus Creator/4  "RotMat2D"
  [TransVec] -> Bus Creator/5  "TranslationVec"
  Bus Selector/2 -> Terminator1/1  "<RadarType>"
  Bus Selector/3 -> Terminator2/1  "<isActive>"
  Bus Selector/4 -> Terminator3/1  "<RotMat2D>"
  Bus Selector/8 -> Bus Creator/8  "<MountZ>"
  Bus Selector/5 -> Terminator4/1  "<TranslationVec>"
  Bus Selector/7 -> Terminator6/1  "<MountY>"
  Bus Selector/6 -> Terminator5/1  "<MountX>"
  Bus Selector/9 -> Terminator8/1  "<MountYaw>"
  Bus Selector/11 -> Bus Creator/11  "<MountRoll>"
  Bus Selector/10 -> Bus Creator/10  "<MountPitch>"
  Selector5/1 -> Bus Creator/12  "nMeas"
  Constant4/1 -> Selector5/1
  Bus Selector/12 -> Terminator7/1  "<nMeas>"

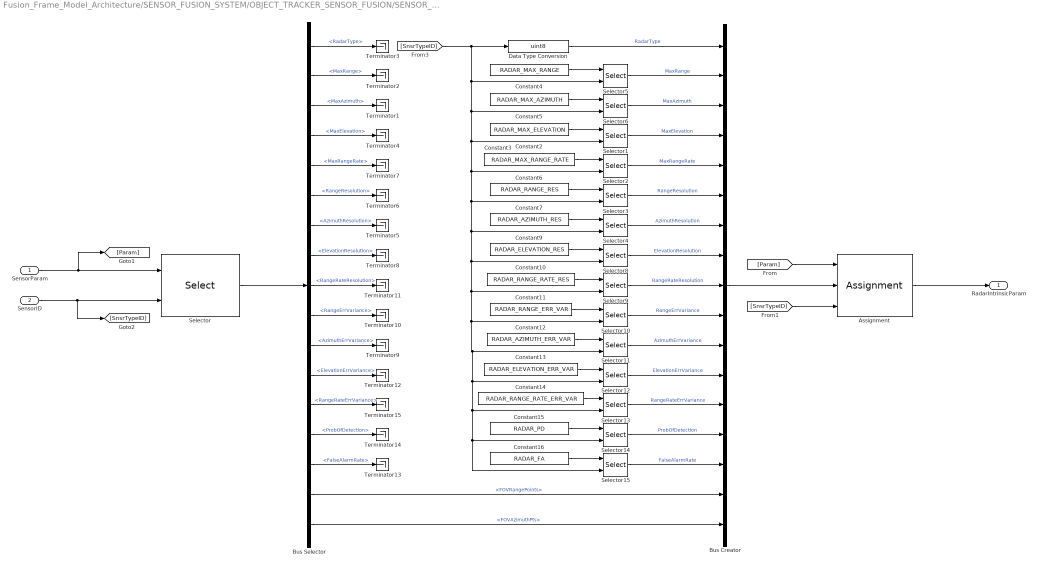
== system Fusion_Frame_Model_Architecture/SENSOR_FUSION_SYSTEM/OBJECT_TRACKER_SENSOR_FUSION/SENSOR_LAYOUT_AND_CHRACTERIZATION/SET_SENSOR_CALLIBRATION_PARAMETER/SET_RADAR_SENSOR_PARAM/SET_RADAR_INTRINSIC_PARAM/SET_RADAR_INTRINSIC_PARAM ==
  SensorParam : Inport
  SensorID : Inport  Port=2
  Assignment : Assignment  DiagnosticForDimensions=Warning  IndexOptions=Index vector (port)  Indices=1  OutputSizes=1
  Bus Creator : BusCreator  Inputs=17  OutDataTypeStr=Bus: RadarIntrinsicParam  NonVirtualBus=on
  Bus Selector : BusSelector  OutputSignals=RadarType,MaxRange,MaxAzimuth,MaxElevation,MaxRangeRate,RangeResolution,AzimuthResolution,ElevationResolution,RangeRateResolution,RangeErrVariance,AzimuthErrVariance,ElevationErrVariance,RangeRateErrVariance,ProbOfDetection,FalseAlarmRate,FOVRangePoints,FOVAzimuthPts
  Constant10 : Constant  Value=RADAR_RANGE_RATE_RES
  Constant11 : Constant  Value=RADAR_RANGE_ERR_VAR
  Constant12 : Constant  Value=RADAR_AZIMUTH_ERR_VAR
  Constant13 : Constant  Value=RADAR_ELEVATION_ERR_VAR
  Constant14 : Constant  Value=RADAR_RANGE_RATE_ERR_VAR
  Constant15 : Constant  Value=RADAR_PD
  Constant16 : Constant  Value=RADAR_FA
  Constant2 : Constant  Value=RADAR_MAX_ELEVATION
  Constant3 : Constant  Value=RADAR_MAX_RANGE_RATE
  Constant4 : Constant  Value=RADAR_MAX_RANGE
  Constant5 : Constant  Value=RADAR_MAX_AZIMUTH
  Constant6 : Constant  Value=RADAR_RANGE_RES
  Constant7 : Constant  Value=RADAR_AZIMUTH_RES
  Constant9 : Constant  Value=RADAR_ELEVATION_RES
  Data Type Conversion : DataTypeConversion  OutDataTypeStr=uint8
  Selector{,1..6,8..15} (15 alike) : Selector  InputPortWidth=nRadarTypes  IndexOptions=Index vector (port)  Indices=[1 3]  OutputSizes=1
  Terminator{1..15} (15 alike) : Terminator
  RadarIntrinsicParam : Outport
  wires:
  Assignment/1 -> RadarIntrinsicParam/1
  SensorParam/1 -> [Param], Selector/1
  Selector/1 -> Bus Selector/1
  Bus Creator/1 -> Assignment/2
  SensorID/1 -> [SnsrTypeID], Selector/2
  [Param] -> Assignment/1
  [SnsrTypeID] -> Assignment/3
  Bus Selector/17 -> Bus Creator/17  "<FOVAzimuthPts>"
  Bus Selector/16 -> Bus Creator/16  "<FOVRangePoints>"
  Constant5/1 -> Selector6/1
  Constant4/1 -> Selector5/1
  Bus Selector/3 -> Terminator1/1  "<MaxAzimuth>"
  Bus Selector/2 -> Terminator2/1  "<MaxRange>"
  Bus Selector/1 -> Terminator3/1  "<RadarType>"
  Selector6/1 -> Bus Creator/3  "MaxAzimuth"
  Selector5/1 -> Bus Creator/2  "MaxRange"
  [SnsrTypeID] -> Selector14/2, Selector15/2, Selector13/2, Selector12/2, Selector11/2, Selector10/2, Selector9/2, Selector8/2, Selector4/2, Selector3/2, Selector2/2, Selector1/2, Selector6/2, Selector5/2, Data Type Conversion/1
  Selector1/1 -> Bus Creator/4  "MaxElevation"
  Selector2/1 -> Bus Creator/5  "MaxRangeRate"
  Selector3/1 -> Bus Creator/6  "RangeResolution"
  Selector4/1 -> Bus Creator/7  "AzimuthResolution"
  Selector8/1 -> Bus Creator/8  "ElevationResolution"
  Constant2/1 -> Selector1/1
  Constant3/1 -> Selector2/1
  Constant6/1 -> Selector3/1
  Constant7/1 -> Selector4/1
  Constant9/1 -> Selector8/1
  Selector9/1 -> Bus Creator/9  "RangeRateResolution"
  Selector10/1 -> Bus Creator/10  "RangeErrVariance"
  Selector11/1 -> Bus Creator/11  "AzimuthErrVariance"
  Selector12/1 -> Bus Creator/12  "ElevationErrVariance"
  Selector13/1 -> Bus Creator/13  "RangeRateErrVariance"
  Selector14/1 -> Bus Creator/14  "ProbOfDetection"
  Selector15/1 -> Bus Creator/15  "FalseAlarmRate"
  Constant10/1 -> Selector9/1
  Constant11/1 -> Selector10/1
  Constant12/1 -> Selector11/1
  Constant13/1 -> Selector12/1
  Constant14/1 -> Selector13/1
  Constant15/1 -> Selector14/1
  Constant16/1 -> Selector15/1
  Bus Selector/4 -> Terminator4/1  "<MaxElevation>"
  Bus Selector/7 -> Terminator5/1  "<AzimuthResolution>"
  Bus Selector/6 -> Terminator6/1  "<RangeResolution>"
  Bus Selector/8 -> Terminator8/1  "<ElevationResolution>"
  Bus Selector/5 -> Terminator7/1  "<MaxRangeRate>"
  Bus Selector/11 -> Terminator9/1  "<AzimuthErrVariance>"
  Bus Selector/14 -> Terminator14/1  "<ProbOfDetection>"
  Bus Selector/10 -> Terminator10/1  "<RangeErrVariance>"
  Bus Selector/13 -> Terminator15/1  "<RangeRateErrVariance>"
  Bus Selector/12 -> Terminator12/1  "<ElevationErrVariance>"
  Bus Selector/15 -> Terminator13/1  "<FalseAlarmRate>"
  Bus Selector/9 -> Terminator11/1  "<RangeRateResolution>"
  Data Type Conversion/1 -> Bus Creator/1  "RadarType"

== system Fusion_Frame_Model_Architecture/SENSOR_FUSION_SYSTEM/OBJECT_TRACKER_SENSOR_FUSION/SPATIAL_ALLIGNMENT1/CAMERA_MEASUREMENTS_SPATIAL_ALLIGNMENT/For Iterator Subsystem/For Iterator Subsystem/CoordinateTransformation1 ==
  meas : Inport
  SensorParam : Inport  Port=2
  Action Port : ActionPort  ActionType=then
  InfoExtractor : Subsystem
  Meas_Noise_Cov_Transformation : Subsystem
  Position_Transformation : Subsystem
  Subsystem : Subsystem
  Velocity_Transformation : Subsystem
  measUpd : Outport
  wires:
  meas/1 -> InfoExtractor/1(In1)
  SensorParam/1 -> InfoExtractor/2(In2)
  Velocity_Transformation/1(VelXcts) -> [VxCTS]  "vxCTS"
  InfoExtractor/5(RotMat2D) -> Velocity_Transformation/3(RotMatrix2D), Meas_Noise_Cov_Transformation/1(RotMatrix), [RotMat]
  InfoExtractor/4(<vy>) -> Velocity_Transformation/2(Vy)
  InfoExtractor/3(<vx>) -> Velocity_Transformation/1(Vx)
  InfoExtractor/1(<px>) -> Position_Transformation/1(Px)
  InfoExtractor/2(<py>) -> Position_Transformation/2(Py)
  InfoExtractor/7(MeasNoiseCov) -> Meas_Noise_Cov_Transformation/2(MeasCovarience)
  [RotMat] -> Position_Transformation/3(RotationMat)
  [TransVector] -> Position_Transformation/4(TranslationVector)
  InfoExtractor/6(TransVec2D) -> [TransVector]
  Position_Transformation/1(PosXcts) -> Subsystem/1(pxCTS)
  Meas_Noise_Cov_Transformation/1(MeasCovTransformed) -> Subsystem/5(covCTS)
  Position_Transformation/2(PosYcts) -> Subsystem/2(pyCTS)
  Velocity_Transformation/2(VelYcts) -> [VyCTS]  "vyCTS"
  [VxCTS] -> Subsystem/3(vxCTS)
  [VyCTS] -> Subsystem/4(vyCTS)
  Subsystem/1(measUpd) -> measUpd/1

== system Fusion_Frame_Model_Architecture/SENSOR_FUSION_SYSTEM/OBJECT_TRACKER_SENSOR_FUSION/SPATIAL_ALLIGNMENT1/CAMERA_MEASUREMENTS_SPATIAL_ALLIGNMENT/For Iterator Subsystem/For Iterator Subsystem/SetMeasurement1 ==
  measTransformed : Inport
  CameraMeasCAN : Inport  Port=2
  measID : Inport  Port=3
  CamCANidx : Inport  Port=4
  Assignment1 : Assignment  NumberOfDimensions=2  DiagnosticForDimensions=Warning  IndexOptions=Assign all,Index vector (port)  Indices=1:2,1  OutputSizes=1,1
  Assignment2 : Assignment  NumberOfDimensions=3  DiagnosticForDimensions=Warning  IndexOptions=Assign all,Assign all,Index vector (port)  Indices=1:8,1,1  OutputSizes=1,1,1
  Assignment3 : Assignment  NumberOfDimensions=2  DiagnosticForDimensions=Warning  IndexOptions=Assign all,Index vector (port)  Indices=1:8,1  OutputSizes=1,1
  Bus Selector : BusSelector  OutputSignals=measID,cameraID
  Bus Selector1 : BusSelector  OutputSignals=stateCTS,covCTS
  Constant : Constant  Value=single(zeros(2,1))
  Constant1 : Constant  Value=single(zeros(2,2))
  Constant2 : Constant  Value=uint16(zeros(2,1))
  Data Type Conversion : DataTypeConversion  OutDataTypeStr=uint16
  Mux : Mux  Inputs=2
  Reshape : Reshape  OutputDimensionality=Column vector (2-D)
  Switch : Switch  Criteria=u2 ~= 0
  Switch1 : Switch  Criteria=u2 ~= 0
  Switch2 : Switch  Criteria=u2 ~= 0
  Unit Delay : UnitDelay  InitialCondition=single(zeros(2, 200))  SampleTime=-1
  Unit Delay1 : UnitDelay  InitialCondition=single(zeros(2, 2, 200))  SampleTime=-1
  Unit Delay2 : UnitDelay  InitialCondition=uint16(zeros(2, 200))  SampleTime=-1
  CameraCTSMatUpd : Outport
  CameraCTSNoiseCovMatUpd : Outport  Port=2
  CameraCTSRefUpd : Outport  Port=3
  wires:
  measID/1 -> Switch/2, Switch2/2, Switch1/2
  Constant/1 -> Switch/3
  Switch/1 -> Assignment1/2
  CamCANidx/1 -> [idx], Assignment1/3
  CameraMeasCAN/1 -> Bus Selector/1
  Unit Delay/1 -> Assignment1/1
  Assignment1/1 -> [CTSMat], CameraCTSMatUpd/1
  Bus Selector/1 -> Mux/1  "<measID>"
  Bus Selector/2 -> Data Type Conversion/1  "<cameraID>"
  Mux/1 -> Reshape/1
  Unit Delay1/1 -> Assignment2/1
  Switch1/1 -> Assignment2/2
  measTransformed/1 -> Bus Selector1/1
  Bus Selector1/1 -> Switch/1  "<stateCTS>"
  Constant1/1 -> Switch1/3
  Bus Selector1/2 -> [CTSNoiseCov]  "<covCTS>"
  [CTSNoiseCov] -> Switch1/1
  [idx] -> Assignment2/3
  Switch2/1 -> Assignment3/2
  Constant2/1 -> Switch2/3
  [idx] -> Assignment3/3
  Unit Delay2/1 -> Assignment3/1
  Reshape/1 -> [CTSRef]
  [CTSRef] -> Switch2/1
  Assignment2/1 -> [CTSMatCov], CameraCTSNoiseCovMatUpd/1
  Assignment3/1 -> [CTSRefMat], CameraCTSRefUpd/1
  Data Type Conversion/1 -> Mux/2
  [CTSRefMat] -> Unit Delay2/1
  [CTSMatCov] -> Unit Delay1/1
  [CTSMat] -> Unit Delay/1

== system Fusion_Frame_Model_Architecture/SENSOR_FUSION_SYSTEM/OBJECT_TRACKER_SENSOR_FUSION/SPATIAL_ALLIGNMENT1/CAMERA_MEASUREMENTS_SPATIAL_ALLIGNMENT/For Iterator Subsystem/For Iterator Subsystem/Subsystem ==
  measCAN : Inport
  measIdx : Inport  Port=2
  Add : Sum
  Bus Selector : BusSelector  OutputSignals=measID
  Constant : Constant  Value=int32(0)
  Constant2 : Constant  Value=int32(1)
  If : If  IfExpression=u1 ~= 0  ShowElse=off
  Selector : Selector  NumberOfDimensions=2  InputPortWidth=3  IndexOptions=Select all,Index vector (port)  Indices=[1 3],1  OutputSizes=1,1
  Switch : Switch  Criteria=u2 ~= 0
  Unit Delay : UnitDelay  InitialCondition=int32(0)  SampleTime=-1
  nValidMeasCnt : Outport
  isValid : Outport  Port=2
  meas_i : Outport  Port=3
  measID : Outport  Port=4
  wires:
  measIdx/1 -> Selector/2
  Selector/1 -> meas_i/1, Bus Selector/1
  measCAN/1 -> Selector/1
  If/1 -> isValid/1
  Switch/1 -> Add/1
  Bus Selector/1 -> measID/1, If/1, Switch/2  "<measID>"
  Constant2/1 -> Switch/1
  Unit Delay/1 -> Add/2
  Constant/1 -> Switch/3
  Add/1 -> nValidMeasCnt/1, Unit Delay/1

== system Fusion_Frame_Model_Architecture/SENSOR_FUSION_SYSTEM/OBJECT_TRACKER_SENSOR_FUSION/SPATIAL_ALLIGNMENT1/RADAR_MEASUREMENTS_SPATIAL_ALLIGNMENT/RADAR_MEASUREMENTS_SPATIAL_ALLIGNMENT/COORDINATE_TRANSFORMATION/COORDINATE_TRANSFORMATION ==
  meas : Inport
  SensorParam : Inport  Port=2
  Action Port : ActionPort  ActionType=then
  GET_DATA : Subsystem
  MEAS_NOISE_COV_TRANSFORMATION : Subsystem
  POSITION_TRANSFORMATION : Subsystem
  SET_DATA : Subsystem
  VELOCITY_TRANSFORMATION : Subsystem
  measUpd : Outport
  wires:
  meas/1 -> GET_DATA/1(In1)
  SensorParam/1 -> GET_DATA/2(In2)
  VELOCITY_TRANSFORMATION/1(VelXcts) -> [VxCTS]  "vxCTS"
  GET_DATA/5(RotMat2D) -> VELOCITY_TRANSFORMATION/3(RotMatrix2D), MEAS_NOISE_COV_TRANSFORMATION/1(RotMatrix), [RotMat]
  GET_DATA/4(<vy>) -> VELOCITY_TRANSFORMATION/2(Vy)
  GET_DATA/3(<vx>) -> VELOCITY_TRANSFORMATION/1(Vx)
  GET_DATA/1(<px>) -> POSITION_TRANSFORMATION/1(Px)
  GET_DATA/2(<py>) -> POSITION_TRANSFORMATION/2(Py)
  GET_DATA/7(MeasNoiseCov) -> MEAS_NOISE_COV_TRANSFORMATION/2(MeasCovarience)
  [RotMat] -> POSITION_TRANSFORMATION/3(RotationMat)
  [TransVector] -> POSITION_TRANSFORMATION/4(TranslationVector)
  GET_DATA/6(TransVec2D) -> [TransVector]
  POSITION_TRANSFORMATION/1(PosXcts) -> SET_DATA/1(pxCTS)
  MEAS_NOISE_COV_TRANSFORMATION/1(MeasCovTransformed) -> SET_DATA/5(covCTS)
  POSITION_TRANSFORMATION/2(PosYcts) -> SET_DATA/2(pyCTS)
  VELOCITY_TRANSFORMATION/2(VelYcts) -> [VyCTS]  "vyCTS"
  [VxCTS] -> SET_DATA/3(vxCTS)
  [VyCTS] -> SET_DATA/4(vyCTS)
  SET_DATA/1(measUpd) -> measUpd/1

== system Fusion_Frame_Model_Architecture/SENSOR_FUSION_SYSTEM/OBJECT_TRACKER_SENSOR_FUSION/SPATIAL_ALLIGNMENT1/RADAR_MEASUREMENTS_SPATIAL_ALLIGNMENT/RADAR_MEASUREMENTS_SPATIAL_ALLIGNMENT/COORDINATE_TRANSFORMATION/GET_DATA ==
  measCAN : Inport
  measIdx : Inport  Port=2
  Add : Sum
  Bus Selector : BusSelector  OutputSignals=measID
  Constant : Constant  Value=int32(0)
  Constant2 : Constant  Value=int32(1)
  If : If  IfExpression=u1 ~= 0  ShowElse=off
  Selector : Selector  NumberOfDimensions=2  InputPortWidth=3  IndexOptions=Select all,Index vector (port)  Indices=[1 3],1  OutputSizes=1,1
  Switch : Switch  Criteria=u2 ~= 0
  Unit Delay : UnitDelay  InitialCondition=int32(0)  SampleTime=-1
  isValid : Outport
  nValidMeasCnt : Outport  Port=2
  meas_i : Outport  Port=3
  measID : Outport  Port=4
  wires:
  measIdx/1 -> Selector/2
  Selector/1 -> meas_i/1, Bus Selector/1
  measCAN/1 -> Selector/1
  If/1 -> isValid/1
  Switch/1 -> Add/1
  Bus Selector/1 -> measID/1, If/1, Switch/2  "<measID>"
  Constant2/1 -> Switch/1
  Unit Delay/1 -> Add/2
  Constant/1 -> Switch/3
  Add/1 -> nValidMeasCnt/1, Unit Delay/1

== system Fusion_Frame_Model_Architecture/SENSOR_FUSION_SYSTEM/OBJECT_TRACKER_SENSOR_FUSION/SPATIAL_ALLIGNMENT1/RADAR_MEASUREMENTS_SPATIAL_ALLIGNMENT/RADAR_MEASUREMENTS_SPATIAL_ALLIGNMENT/COORDINATE_TRANSFORMATION/SET_DATA ==
  measTransformed : Inport
  RadarMeasCAN : Inport  Port=2
  measID : Inport  Port=3
  RadCANidx : Inport  Port=4
  Assignment1 : Assignment  NumberOfDimensions=2  DiagnosticForDimensions=Warning  IndexOptions=Assign all,Index vector (port)  Indices=1:2,1  OutputSizes=1,1
  Assignment2 : Assignment  NumberOfDimensions=3  DiagnosticForDimensions=Warning  IndexOptions=Assign all,Assign all,Index vector (port)  Indices=1:8,1,1  OutputSizes=1,1,1
  Assignment3 : Assignment  NumberOfDimensions=2  DiagnosticForDimensions=Warning  IndexOptions=Assign all,Index vector (port)  Indices=1:8,1  OutputSizes=1,1
  Bus Selector : BusSelector  OutputSignals=measID,radarID
  Bus Selector1 : BusSelector  OutputSignals=stateCTS,covCTS
  Constant : Constant  Value=single(zeros(2,1))
  Constant1 : Constant  Value=single(zeros(2,2))
  Constant2 : Constant  Value=uint16(zeros(2,1))
  Data Type Conversion : DataTypeConversion  OutDataTypeStr=uint16
  Mux : Mux  Inputs=2
  Reshape : Reshape  OutputDimensionality=Column vector (2-D)
  Switch : Switch  Criteria=u2 ~= 0
  Switch1 : Switch  Criteria=u2 ~= 0
  Switch2 : Switch  Criteria=u2 ~= 0
  Unit Delay : UnitDelay  InitialCondition=single(zeros(2, 200))  SampleTime=-1
  Unit Delay1 : UnitDelay  InitialCondition=single(zeros(2, 2, 200))  SampleTime=-1
  Unit Delay2 : UnitDelay  InitialCondition=uint16(zeros(2, 200))  SampleTime=-1
  RadarCTSMatUpd : Outport
  RadarCTSNoiseCovMatUpd : Outport  Port=2
  RadarCTSRefUpd : Outport  Port=3
  wires:
  measID/1 -> Switch/2, Switch2/2, Switch1/2
  Constant/1 -> Switch/3
  Switch/1 -> Assignment1/2
  RadCANidx/1 -> [idx], Assignment1/3
  RadarMeasCAN/1 -> Bus Selector/1
  Unit Delay/1 -> Assignment1/1
  Assignment1/1 -> [CTSMat], RadarCTSMatUpd/1
  Bus Selector/1 -> Mux/1  "<measID>"
  Bus Selector/2 -> Data Type Conversion/1  "<radarID>"
  Mux/1 -> Reshape/1
  Unit Delay1/1 -> Assignment2/1
  Switch1/1 -> Assignment2/2
  measTransformed/1 -> Bus Selector1/1
  Bus Selector1/1 -> Switch/1  "<stateCTS>"
  Constant1/1 -> Switch1/3
  Bus Selector1/2 -> [CTSNoiseCov]  "<covCTS>"
  [CTSNoiseCov] -> Switch1/1
  [idx] -> Assignment2/3
  Switch2/1 -> Assignment3/2
  Constant2/1 -> Switch2/3
  [idx] -> Assignment3/3
  Unit Delay2/1 -> Assignment3/1
  Reshape/1 -> [CTSRef]
  [CTSRef] -> Switch2/1
  Assignment2/1 -> [CTSMatCov], RadarCTSNoiseCovMatUpd/1
  Assignment3/1 -> [CTSRefMat], RadarCTSRefUpd/1
  Data Type Conversion/1 -> Mux/2
  [CTSMat] -> Unit Delay/1
  [CTSMatCov] -> Unit Delay1/1
  [CTSRefMat] -> Unit Delay2/1

== system Fusion_Frame_Model_Architecture/SENSOR_FUSION_SYSTEM/OBJECT_TRACKER_SENSOR_FUSION/CAMERA_HOMOGENEOUS_FUSION/NEAREST_NEIGHBOUR_CLUSTERING_FOR_CAMERA_MEASUREMENT/NN_MEASUREMENT_GROUPING_WITHIN_EPS/For Iterator Subsystem/NN/PERFORM_NN_CLUSTERING ==
  nMeas : Inport
  measArray : Inport  Port=2
  CLSTR_DATA : Inport  Port=3
  idx_i : Inport  Port=4
  CHECK_CONDITION : Subsystem
  For Iterator : ForIterator  ResetStates=reset  IterationSource=external
  SET_DATA : Subsystem
  CLSTR_DATA_UPD : Outport  OutDataTypeStr=Bus: CLUSTER_DATA_STRUCT_SNSR
  wires:
  nMeas/1 -> For Iterator/1
  idx_i/1 -> CHECK_CONDITION/2(idx_i)
  measArray/1 -> CHECK_CONDITION/1(MEAS)
  For Iterator/1 -> [y_j], CHECK_CONDITION/3(idx_j)
  CHECK_CONDITION/1(isMember) -> SET_DATA/1(isClusterMember)
  SET_DATA/1(CLSTR_DATA_UPD) -> CHECK_CONDITION/5(CLSTR_DATA_PREV), CLSTR_DATA_UPD/1
  CLSTR_DATA/1 -> CHECK_CONDITION/4(CLSTR_DATA_INIT)
  CHECK_CONDITION/2(CLSTR_DATA) -> SET_DATA/2(CLSTR_DATA)
  [y_j] -> SET_DATA/3(idx_j)

== system Fusion_Frame_Model_Architecture/SENSOR_FUSION_SYSTEM/OBJECT_TRACKER_SENSOR_FUSION/CAMERA_HOMOGENEOUS_FUSION/NEAREST_NEIGHBOUR_CLUSTERING_FOR_CAMERA_MEASUREMENT/NN_MEASUREMENT_GROUPING_WITHIN_EPS/For Iterator Subsystem/NN/SET_CLUSTER_ID_AND_UPDATE_NUMBER_OF_CLUSTERS ==
  CLUSTERING_DATA : Inport
  CAM_MEAS_CTS : Inport  Port=2
  Add2 : Sum
  Bus Creator : BusCreator  Inputs=7  OutDataTypeStr=Bus: CLUSTER_DATA_STRUCT_SNSR  NonVirtualBus=on
      settings: InheritFromInputs=off
  Bus Selector : BusSelector  OutputSignals=nClusters
  Bus Selector1 : BusSelector  OutputSignals=ValidCumulativeMeasCount
  Bus Selector2 : BusSelector  OutputSignals=ClusterCenter,ClusterCovariance,ClusterSizes,ClusterToMeasAssignment,isMeasVisitedFlag,nClusters,ClusterMember
  Constant3 : Constant  Value=uint16(1)
  Data Type Conversion : DataTypeConversion  OutDataTypeStr=uint16
  Selector : Selector  NumberOfDimensions=2  InputPortWidth=3  IndexOptions=Select all,Index vector (port)  Indices=[1 3],1  OutputSizes=1,1
  Terminator1 : Terminator
  Width : Width
  nRadMeas : Outport
  CLUSTER_DATA : Outport  Port=2
  wires:
  CLUSTERING_DATA/1 -> Bus Selector2/1, Bus Selector/1
  Bus Selector/1 -> Add2/1  "<nClusters>"
  CAM_MEAS_CTS/1 -> Bus Selector1/1
  Add2/1 -> Data Type Conversion/1
  Constant3/1 -> Add2/2
  Data Type Conversion/1 -> [B]
  Bus Selector2/1 -> Bus Creator/1  "<ClusterCenter>"
  Bus Selector2/2 -> Bus Creator/2  "<ClusterCovariance>"
  Bus Selector2/3 -> Bus Creator/3  "<ClusterSizes>"
  Bus Selector2/4 -> Bus Creator/4  "<ClusterToMeasAssignment>"
  Bus Selector2/5 -> Bus Creator/5  "<isMeasVisitedFlag>"
  Bus Selector2/7 -> Bus Creator/7  "<ClusterMember>"
  Bus Selector2/6 -> Terminator1/1  "<nClusters>"
  [B] -> Bus Creator/6  "nClusters"
  Bus Creator/1 -> CLUSTER_DATA/1
  Bus Selector1/1 -> Width/1, Selector/1  "<ValidCumulativeMeasCount>"
  Width/1 -> Selector/2
  Selector/1 -> nRadMeas/1

== system Fusion_Frame_Model_Architecture/SENSOR_FUSION_SYSTEM/OBJECT_TRACKER_SENSOR_FUSION/CAMERA_HOMOGENEOUS_FUSION/NEAREST_NEIGHBOUR_CLUSTERING_FOR_CAMERA_MEASUREMENT/NN_MEASUREMENT_GROUPING_WITHIN_EPS/For Iterator Subsystem/NN/Subsystem ==
  CLSTR_DATA : Inport
  Bus Selector : BusSelector  OutputSignals=ClusterSizes,nClusters
  Selector : Selector  NumberOfDimensions=2  InputPortWidth=3  IndexOptions=Select all,Index vector (port)  Indices=[1 3],1  OutputSizes=1,1
  ClstrSize : Outport
  wires:
  Bus Selector/2 -> Selector/2  "<nClusters>"
  Bus Selector/1 -> Selector/1  "<ClusterSizes>"
  CLSTR_DATA/1 -> Bus Selector/1
  Selector/1 -> ClstrSize/1
